simulink model "PIFilter"  (R2024b)
settings: Solver=VariableStepAuto  StartTime=0.0  StopTime=0.5  FixedStep=1e9  RelTol=1e-3
values from neighbouring files (symbols this model uses):
  params = struct()    [initialize_noise_parameters.m]
libraries: fl_lib x19, ee_lib x6, nesl_utility x6
settings Model: Creator=const  LastModifiedBy=const
settings SolverCC: ZeroCrossAlgorithm=Adaptive

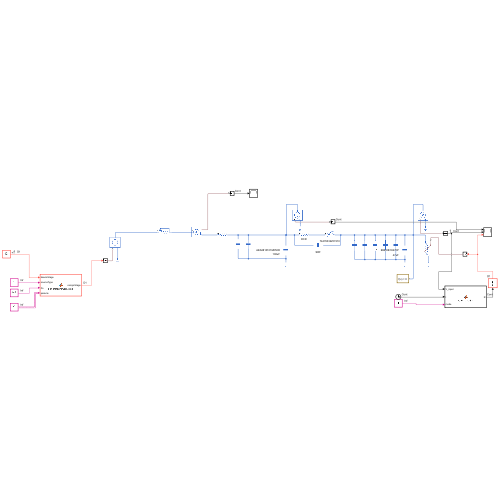
[thumbnail: Simulink's stored preview of the top-level diagram]
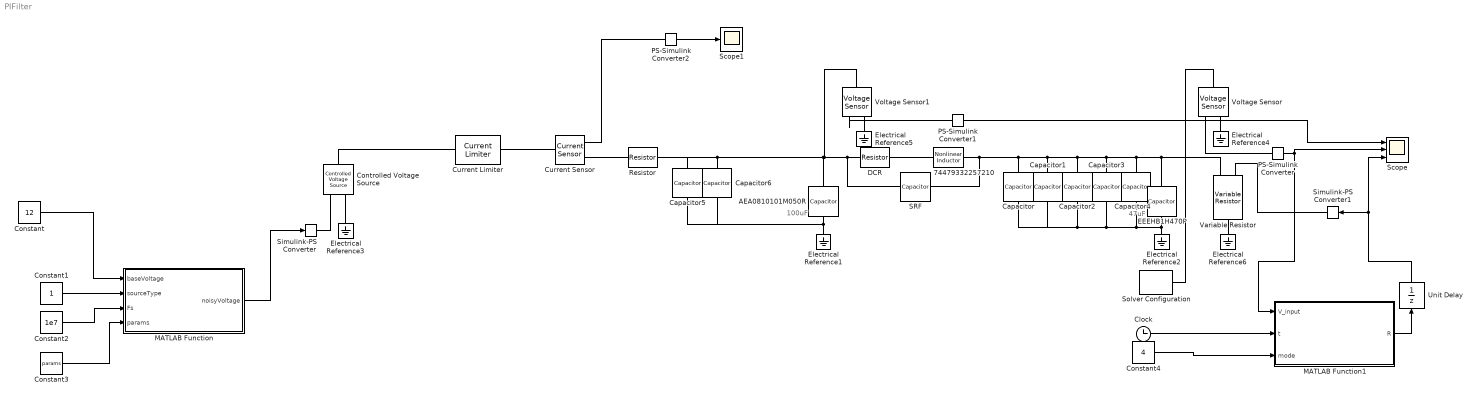
== system PIFilter ==
  note: 100uF
  note: 47uF
  74479332257210 : ee_lib/Passive/Nonlinear Inductor  parameterization_option=3  Nw=10  L=2e-4 H  L_sat=1e-4 H  current_data=[0, 2, 4, 6, 8, 10] A  magnetic_flux_data=[0, 2, 3.95, 5.75, 7.35, 8.77] .* 1e-5 Wb  H_data=[0, 200, 400, 600, 800, 1000] A/m  B_data=[0, .81, 1.25, 1.42, 1.48, 1.49] T  magnetic_flux_sat=1.3e-05 Wb  length_effective=0.032 m  area_effective=1.6e-5 m^2  dBdH0=0.005 T*m/A  B1=1.49 T  H1=1000 A/m  c=0.1  K=200 A/m  alpha=1e-4  averaging_period=0 s  G_parasitic=1e-9 1/Ohm  interpolation_option=1  x0_option=1  i_L0=0 A  phi0=0 Wb  B0=0 T  H0=0 A/m
      settings: InternalSimscapePortConfiguration="{\"Bottom\":[],\"Left\":[{\"id\":\"p\",\"label\":\"+\",\"type\":\"foundation.electrical.electrical\"}],\"Right\":[{\"id\":\"n\",\"label\":\"-\",\"type\":\"foundation.electrical.electrical\"}],\"Top\":[]}"
  AEA0810101M050R : ee_lib/Passive/Capacitor  cap_option=ee.enum.passive.capacitor.capOption.const  c=100e-6 F  Cvec=[1e-05, 1e-06] F  Vvec=[0, 10] V  CV_table_symmetry=ee.enum.passive.capacitor.tableSymmetry.yes  f_vec=[1, 10] kHz  DFext_vec=[.8, 1.2]  enable_C_tol=ee.enum.toleranceApplication.applyRand  averaging_period=0 s  C_tol=20  tol_distribution=ee.enum.toleranceDistribution.uniform  nSigma=4  r=0.34 Ohm  g=1e-6 1/Ohm  enable_operating_limits=ee.enum.enable.yes  operating_limit_action=ee.enum.passive.reportOpLim.warn  max_working_voltage_range=[0, 50] V  power_rating=0.037 W  maxTemperature=105 degC  thermalEnable=false  thermalMass=1 J/K  fault_action=simscape.enum.assert.action.none  t_fault=1 s  i_specify=off  i_priority=None  i=0 A  i_nominal_specify=off  i_nominal_value=1  i_nominal_unit=A  v_specify=off  v_priority=None  v=0 V  v_nominal_specify=off  v_nominal_value=1  v_nominal_unit=V  vc_specify=off  vc_priority=High  vc=0 V  vc_nominal_specify=off  vc_nominal_value=1  vc_nominal_unit=V  T_specify=off  T_priority=None  T=298.15 K  T_nominal_specify=off  T_nominal_value=1  T_nominal_unit=K
  Capacitor{,1..2,5..6} (5 alike) : fl_lib/Electrical/Electrical Elements/Capacitor  c=10 uF  r=1e-6 Ohm  g=0 1/Ohm  i_specify=off  i_priority=None  i=0 A  i_nominal_specify=off  i_nominal_value=1  i_nominal_unit=A  v_specify=off  v_priority=None  v=0 V  v_nominal_specify=off  v_nominal_value=1  v_nominal_unit=V  vc_specify=off  vc_priority=High  vc=0 V  vc_nominal_specify=off  vc_nominal_value=1  vc_nominal_unit=V
  Capacitor3 : fl_lib/Electrical/Electrical Elements/Capacitor  c=4.7 uF  r=1e-6 Ohm  g=0 1/Ohm  i_specify=off  i_priority=None  i=0 A  i_nominal_specify=off  i_nominal_value=1  i_nominal_unit=A  v_specify=off  v_priority=None  v=0 V  v_nominal_specify=off  v_nominal_value=1  v_nominal_unit=V  vc_specify=off  vc_priority=High  vc=0 V  vc_nominal_specify=off  vc_nominal_value=1  vc_nominal_unit=V
  Capacitor4 : fl_lib/Electrical/Electrical Elements/Capacitor  c=2.2 uF  r=1e-6 Ohm  g=0 1/Ohm  i_specify=off  i_priority=None  i=0 A  i_nominal_specify=off  i_nominal_value=1  i_nominal_unit=A  v_specify=off  v_priority=None  v=0 V  v_nominal_specify=off  v_nominal_value=1  v_nominal_unit=V  vc_specify=off  vc_priority=High  vc=0 V  vc_nominal_specify=off  vc_nominal_value=1  vc_nominal_unit=V
  Clock : Clock
  Constant : Constant  Value=12  SampleTime=1e-6
  Constant1 : Constant
  Constant2 : Constant  Value=1e7
  Constant3 : Constant  Value=params  OutDataTypeStr=Bus: paramsBus
  Constant4 : Constant  Value=4
  Controlled Voltage Source : fl_lib/Electrical/Electrical Sources/Controlled Voltage Source
  Current Limiter : ee_lib/Semiconductors & Converters/Current Limiter  limType=ee.enum.semiconductors.currLimType.constLim  iLim=3 A  iLimReverse=1 A  vLim=0.01 V  gLim=1e-3 1/Ohm  thermal_mass=100 J/K  temperature_specify=off  temperature_priority=High  temperature=298.15 K  temperature_nominal_specify=off  temperature_nominal_value=1  temperature_nominal_unit=K
      settings: InternalSimscapePortConfiguration="{\"Bottom\":[],\"Left\":[{\"id\":\"p\",\"label\":\"+\",\"type\":\"foundation.electrical.electrical\"}],\"Right\":[{\"id\":\"n\",\"label\":\"-\",\"type\":\"foundation.electrical.electrical\"}],\"Top\":[]}"
  Current Sensor : fl_lib/Electrical/Electrical Sensors/Current Sensor
  DCR : fl_lib/Electrical/Electrical Elements/Resistor  R=23.3 mOhm  i_specify=off  i_priority=None  i=0 A  i_nominal_specify=off  i_nominal_value=1  i_nominal_unit=A  v_specify=off  v_priority=None  v=0 V  v_nominal_specify=off  v_nominal_value=1  v_nominal_unit=V
  EEEHB1H470P : ee_lib/Passive/Capacitor  cap_option=ee.enum.passive.capacitor.capOption.const  c=47e-6 F  Cvec=[1e-05, 1e-06] F  Vvec=[0, 10] V  CV_table_symmetry=ee.enum.passive.capacitor.tableSymmetry.yes  f_vec=[1, 10] kHz  DFext_vec=[.8, 1.2]  enable_C_tol=ee.enum.toleranceApplication.applyRand  averaging_period=0 s  C_tol=20  tol_distribution=ee.enum.toleranceDistribution.uniform  nSigma=4  r=0.4 Ohm  g=0.47e-6 1/Ohm  enable_operating_limits=ee.enum.enable.yes  operating_limit_action=ee.enum.passive.reportOpLim.warn  max_working_voltage_range=[0, 50] V  power_rating=0.0338 W  maxTemperature=85 degC  thermalEnable=false  thermalMass=1 J/K  fault_action=simscape.enum.assert.action.none  t_fault=1 s  i_specify=off  i_priority=None  i=0 A  i_nominal_specify=off  i_nominal_value=1  i_nominal_unit=A  v_specify=off  v_priority=None  v=0 V  v_nominal_specify=off  v_nominal_value=1  v_nominal_unit=V  vc_specify=off  vc_priority=High  vc=0 V  vc_nominal_specify=off  vc_nominal_value=1  vc_nominal_unit=V  T_specify=off  T_priority=None  T=298.15 K  T_nominal_specify=off  T_nominal_value=1  T_nominal_unit=K
  Electrical Reference{1..6} (6 alike) : fl_lib/Electrical/Electrical Elements/Electrical Reference
  MATLAB Function : MATLAB Function  TreatAsAtomicUnit=on
  MATLAB Function1 : MATLAB Function  TreatAsAtomicUnit=on
  PS-Simulink Converter : nesl_utility/PS-Simulink Converter  PhysicalDomain=network_engine_domain  SubClassName=ps_output  LeftPortType=input  RightPortType=output  PseudoPeriodic=off  Frequencies=[]  VectorFormat=inherit  Unit=inherit  AffineConversion=off
  PS-Simulink Converter1 : nesl_utility/PS-Simulink Converter  PhysicalDomain=network_engine_domain  SubClassName=ps_output  LeftPortType=input  RightPortType=output  PseudoPeriodic=off  Frequencies=[]  VectorFormat=inherit  Unit=inherit  AffineConversion=off
  PS-Simulink Converter2 : nesl_utility/PS-Simulink Converter  PhysicalDomain=network_engine_domain  SubClassName=ps_output  LeftPortType=input  RightPortType=output  PseudoPeriodic=off  Frequencies=[]  VectorFormat=inherit  Unit=inherit  AffineConversion=off
  Resistor : ee_lib/Passive/Resistor  R=30 mOhm  enable_R_tol=ee.enum.toleranceApplication.applyRand  R_tol=1  tol_distribution=ee.enum.toleranceDistribution.uniform  nSigma=4  enable_operating_limits=ee.enum.enable.no  operating_limit_action=ee.enum.passive.reportOpLim.warn  power_rating=1 W  max_working_voltage=100 V  noise_mode=ee.enum.sources.noise.Disabled  Tdevice=25 degC  sample_time=1e-3 s  repeatability=ee.enum.ic.repeatability.notRepeatable  user_seed=0  auto_seed=686172465  fault_action=simscape.enum.assert.action.none  t_fault=1 s  power_derating_T1=70 degC  power_derating_T2=155 degC  operating_temperature_range_vec=[-50, 150] degC  alpha=3.93e-3 1/K  Tmeas=25 degC  thermal_mass=100 J/K  temperature_specify=off  temperature_priority=High  temperature=298.15 K  temperature_nominal_specify=off  temperature_nominal_value=1  temperature_nominal_unit=K
  SRF : ee_lib/Passive/Capacitor  cap_option=ee.enum.passive.capacitor.capOption.const  c=5.6 pF  Cvec=[1e-05, 1e-06] F  Vvec=[0, 10] V  CV_table_symmetry=ee.enum.passive.capacitor.tableSymmetry.yes  f_vec=[1, 10] kHz  DFext_vec=[.8, 1.2]  enable_C_tol=ee.enum.toleranceApplication.none  averaging_period=0 s  C_tol=5  tol_distribution=ee.enum.toleranceDistribution.uniform  nSigma=4  r=0 Ohm  g=0 1/Ohm  enable_operating_limits=ee.enum.enable.no  operating_limit_action=ee.enum.passive.reportOpLim.warn  max_working_voltage_range=[-25, 25] V  power_rating=1 W  maxTemperature=85 degC  thermalEnable=false  thermalMass=1 J/K  fault_action=simscape.enum.assert.action.none  t_fault=1 s  i_specify=off  i_priority=None  i=0 A  i_nominal_specify=off  i_nominal_value=1  i_nominal_unit=A  v_specify=off  v_priority=None  v=0 V  v_nominal_specify=off  v_nominal_value=1  v_nominal_unit=V  vc_specify=off  vc_priority=High  vc=0 V  vc_nominal_specify=off  vc_nominal_value=1  vc_nominal_unit=V  T_specify=off  T_priority=None  T=298.15 K  T_nominal_specify=off  T_nominal_value=1  T_nominal_unit=K
  Scope : Scope  NumInputPorts=3
  Scope1 : Scope
  Simulink-PS Converter : nesl_utility/Simulink-PS Converter  PhysicalDomain=network_engine_domain  SubClassName=ps_input  LeftPortType=input  RightPortType=output  PseudoPeriodic=off  Frequencies=[]  NoiseDistribution=none  NoiseParameters=[]  Unit=1  AffineConversion=off  FilteringAndDerivatives=filter  SimscapeFilterOrder=1  InputFilterTimeConstant=1e-6  UdotUserProvided=0
  Simulink-PS Converter1 : nesl_utility/Simulink-PS Converter  PhysicalDomain=network_engine_domain  SubClassName=ps_input  LeftPortType=input  RightPortType=output  PseudoPeriodic=off  Frequencies=[]  NoiseDistribution=none  NoiseParameters=[]  Unit=1  AffineConversion=off  FilteringAndDerivatives=provide  SimscapeFilterOrder=1  InputFilterTimeConstant=0.001  UdotUserProvided=0
  Solver Configuration : nesl_utility/Solver Configuration  PhysicalDomain=network_engine_domain  SubClassName=solver  LeftPortType=input  RightPortType=generic  Tones=[]  Harmonics=[]  SimulateNoise=off  Profile=off  UseLocalSampling=off  EnableSwitchedLinearOptims=on  FrequencyDomain=off  UseCCode=off  RelTol=0.001  AbsTol=0.001  MinStep=1e-09  ToWorkspace=off  RevertToSquareIcSolve=off  NumHomotopyIterations=100  PhasorMode=off  PhasorModeNumHarmonics=1  ConsistencySolver=NEWTON_XTOL_AFTER_FTOL  IndexReductionMethod=DerivativeReplacement  DoDC=off  ResidualTolerance=1e-09  ConsistencyTolSource=GLOBAL  ConsistencyAbsTol=0.001  ConsistencyRelTol=0.001  ConsistencyTolFactor=0.001  UseLocalSolver=off  LocalSolverChoice=NE_BACKWARD_EULER_ADVANCER  ResolveIndetEquations=on  FunctionEvalNumThread=1  LocalSolverSampleTime=0.001  DoFixedCost=off  MaxNonlinIter=3  MaxModeIter=2  ComputeImpulses=off  ImpulseIterations=2  LinearAlgebra=auto  LinearAlgebraNumThread=0  EquationFormulation=NE_TIME_EF  DelaysMemoryBudget=1024  AutomaticFiltering=on  FilteringTimeConstant=0.001  PartitionStorageMethod=AS_NEEDED  PartitionMemoryBudget=1024  PartitionMethod=ROBUST  MultibodyUseLocalSolver=off  MultibodyLocalSolverChoice=ODE1  MultibodyLocalSolverSampleTime=0.001
  Unit Delay : UnitDelay  SampleTime=-1  HasFrameUpgradeWarning=on
  Variable Resistor : fl_lib/Electrical/Electrical Elements/Variable Resistor  Rmin=1 Ohm  thermalEnable=false  thermal_mass=1 J/K  i_specify=off  i_priority=None  i=0 A  i_nominal_specify=off  i_nominal_value=1  i_nominal_unit=A  v_specify=off  v_priority=None  v=0 V  v_nominal_specify=off  v_nominal_value=1  v_nominal_unit=V  T_specify=off  T_priority=None  T=300 K  T_nominal_specify=off  T_nominal_value=1  T_nominal_unit=K
  Voltage Sensor : fl_lib/Electrical/Electrical Sensors/Voltage Sensor
  Voltage Sensor1 : fl_lib/Electrical/Electrical Sensors/Voltage Sensor
  wires:
  PS-Simulink Converter/1 -> MATLAB Function1/1(V_input), Scope/2
  Constant/1 -> MATLAB Function/1(baseVoltage)
  PS-Simulink Converter1/1 -> Scope/1
  PS-Simulink Converter2/1 -> Scope1/1
  Constant1/1 -> MATLAB Function/2(sourceType)
  Constant2/1 -> MATLAB Function/3(Fs)
  Constant3/1 -> MATLAB Function/4(params)
  MATLAB Function/1(noisyVoltage) -> Simulink-PS Converter/1
  Constant4/1 -> MATLAB Function1/3(mode)
  Clock/1 -> MATLAB Function1/2(t)
  MATLAB Function1/1(R) -> Unit Delay/1
  Unit Delay/1 -> Scope/3, Simulink-PS Converter1/1
  connections:
  DCR/RConn1 -- 74479332257210/LConn1
  EEEHB1H470P/LConn1 -- Solver Configuration/RConn1 -- Variable Resistor/LConn2 -- Voltage Sensor/LConn1 -- Capacitor4/LConn1 -- Capacitor3/LConn1 -- Capacitor2/LConn1 -- Capacitor1/LConn1 -- Capacitor/LConn1 -- SRF/RConn1 -- 74479332257210/RConn1
  Electrical Reference1/LConn1 -- Capacitor6/RConn1 -- Capacitor5/RConn1 -- AEA0810101M050R/RConn1
  Electrical Reference2/LConn1 -- Capacitor4/RConn1 -- Capacitor3/RConn1 -- Capacitor2/RConn1 -- Capacitor1/RConn1 -- Capacitor/RConn1 -- EEEHB1H470P/RConn1
  AEA0810101M050R/LConn1 -- Resistor/RConn1 -- Capacitor5/LConn1 -- Capacitor6/LConn1 -- DCR/LConn1 -- SRF/LConn1 -- Voltage Sensor1/LConn1
  Electrical Reference3/LConn1 -- Controlled Voltage Source/RConn2
  Electrical Reference4/LConn1 -- Voltage Sensor/RConn2
  Electrical Reference5/LConn1 -- Voltage Sensor1/RConn2
  Variable Resistor/RConn1 -- Electrical Reference6/LConn1
  Voltage Sensor/RConn1 -- PS-Simulink Converter/LConn1
  Simulink-PS Converter/RConn1 -- Controlled Voltage Source/RConn1
  Voltage Sensor1/RConn1 -- PS-Simulink Converter1/LConn1
  PS-Simulink Converter2/LConn1 -- Current Sensor/RConn1
  Current Limiter/RConn1 -- Current Sensor/LConn1
  Current Limiter/LConn1 -- Controlled Voltage Source/LConn1
  Simulink-PS Converter1/RConn1 -- Variable Resistor/LConn1
  Current Sensor/RConn2 -- Resistor/LConn1

== matlab function PIFilter/MATLAB Function1 ==
  data: V_input input; R output; t input; mode input
function R = motorLoadSim(V_input, t, mode)
% MOTORLOADSIM Simulink-compatible DC motor load resistance simulator
%
% Inputs:
%   V_input - Supply voltage (V)
%   t       - Current time (seconds) - scalar input from Simulink Clock
%   mode    - Load pattern: 1=steps, 2=triangles, 3=random, 4=mixed
%
% Output:
%   R - Resistance value (ohms) to achieve desired current profile
%
% Motor specs: Max current = 3A

    % Generate current based on mode
    if mode == 1
        % Steps - sharp step changes
        step_levels = [0.3, 1.0, 0.5, 2.0, 0.8, 2.5, 0.4, 3.0];
        step_duration = 0.5;
        idx = floor(t / step_duration) + 1;
        if idx > 8
            idx = mod(idx-1, 8) + 1;
        end
        I_motor = step_levels(idx);
        
    elseif mode == 2
        % Triangles
        freq = 0.5;
        I_min = 0.2;
        I_max = 3.0;
        phase = mod(freq * t, 1.0);
        if phase < 0.5
            I_motor = I_min + (I_max - I_min) * (phase * 2);
        else
            I_motor = I_max - (I_max - I_min) * ((phase - 0.5) * 2);
        end
        
    elseif mode == 3
        % Random-like (deterministic based on time)
        current_levels = [0.3, 0.8, 1.5, 2.2, 2.8, 3.0, 0.5, 1.2];
        idx = floor(mod(t * 3.7, 8)) + 1; % Pseudo-random indexing
        I_motor = current_levels(idx);
        
    else
        % Mixed pattern (mode == 4 or default)
        cycle_time = 20.0; % 20 second full cycle
        t_phase = mod(t, cycle_time) / cycle_time;
        
        if t_phase < 0.25
            % Step pattern
            I_motor = 0.5 + 2.0 * double(mod(t, 0.3) > 0.15);
            
        elseif t_phase < 0.5
            % Triangle
            tri_phase = mod((t_phase - 0.25) * 8, 1.0);
            if tri_phase < 0.5
                I_motor = 0.3 + 2.7 * (tri_phase * 2);
            else
                I_motor = 3.0 - 2.7 * ((tri_phase - 0.5) * 2);
            end
            
        elseif t_phase < 0.75
            % Spikes
            if mod(floor(t * 10), 3) == 0
                I_motor = 3.0;
            else
                I_motor = 0.4;
            end
            
        else
            % Ramp up
            I_motor = 0.3 + 2.7 * ((t_phase - 0.75) / 0.25);
        end
    end
    
    % Clamp current to valid range
    I_motor = max(min(I_motor, 3.0), 0.2);
    
    % Calculate resistance from Ohm's law
    R = V_input / I_motor;
    
    % Clamp resistance to reasonable values
    R = max(min(R, 1000), 0.1);
end

% Simulink Setup Instructions:
% 1. Add MATLAB Function block
% 2. Copy this entire function into the block
% 3. Inputs: V_input (constant), t (from Clock block), mode (constant 1-4)
% 4. Output: R (connect to your varistor model)
% 5. Set Fixed-step solver (e.g., 0.001s for smooth transitions)

== matlab function PIFilter/MATLAB Function ==
  data: baseVoltage input; noisyVoltage output; sourceType input; Fs input; params input
function noisyVoltage = generatePowerNoise(baseVoltage, sourceType, Fs, params)
% generatePowerNoise - Injects realistic electrical noise onto a base voltage signal.
% OPTIMIZED FOR REAL-TIME SIMULINK PERFORMANCE
%
% Syntax:
%   noisyVoltage = generatePowerNoise(baseVoltage, sourceType, Fs, params)
%
% Inputs:
%   baseVoltage - Scalar or vector representing the ideal, noise-free DC voltage.
%   sourceType  - Scalar: 1=usb_pd, 2=li_po, 3=wall_wart, 0=random
%   Fs          - Scalar: Sampling frequency in Hz.
%   params      - Struct: Contains all configurable parameters for each model.
%
% Output:
%   noisyVoltage - Scalar/vector representing the base voltage with noise superimposed.

    % --- Declare extrinsic functions at the top level ---
    coder.extrinsic('fprintf');

    % --- Handle scalar or vector input ---
    isScalar = isscalar(baseVoltage);
    if isScalar
        baseVoltage = baseVoltage(1);
        len = 1;
    else
        len = length(baseVoltage);
    end
    
    % --- Pre-initialize the noise variable ---
    noise = 0;
    
    % --- Convert sourceType to numeric if needed ---
    sourceTypeNum = sourceType;

    % --- Random Source Selection (only once, not every call) ---
    persistent randomSource
    if isempty(randomSource)
        randomSource = 1;
    end
    
    if sourceTypeNum == 0
        sourceTypeNum = randomSource;
        if rand() < 0.01  % Only change source 1% of the time
            randomSource = randi(3);
            fprintf('Switched to source type: %d\n', randomSource);
        end
    end

    % --- Main Dispatcher ---
    if sourceTypeNum == 1
        % USB PD
        noise = generateUsbPdNoise(baseVoltage, Fs, params.usb_pd, len);
    elseif sourceTypeNum == 2
        % Li-Po
        noise = generateLiPoNoise(baseVoltage, Fs, params.li_po, len);
    elseif sourceTypeNum == 3
        % Wall-Wart
        noise = generateWallWartNoise(baseVoltage, Fs, params.wall_wart, len);
    else
        noise = 0;
    end

    % --- Combine base voltage with generated noise ---
    noisyVoltage = baseVoltage + noise;

end

% --- Sub-function for USB PD Noise ---
function noise = generateUsbPdNoise(baseVoltage, Fs, p, len)
    persistent phase_ripple phase_whine hf_state
    
    % Initialize persistent variables
    if isempty(phase_ripple)
        phase_ripple = 0;
        phase_whine = 0;
        hf_state = 0;
    end
    
    dt = 1/Fs;
    
    % Component 1: Simplified High-Frequency Noise (IIR filtered white noise)
    % Much faster than FFT - uses first-order IIR filter
    if Fs >= 2 * 300e6
        white = randn() * sqrt(p.psd_hf * Fs);
        alpha = 0.95; % Filter coefficient for ~100MHz bandwidth approximation
        hf_state = alpha * hf_state + (1-alpha) * white;
        hf_noise = hf_state;
    else
        hf_noise = 0;
    end
    
    % Component 2: Low-Frequency Ripple and Whine (phase accumulator method)
    % Update phases
    phase_ripple = phase_ripple + 2*pi*p.f_sw*dt;
    phase_whine = phase_whine + 2*pi*p.f_whine*dt;
    
    % Wrap phases to [0, 2*pi] to prevent overflow
    phase_ripple = mod(phase_ripple, 2*pi);
    phase_whine = mod(phase_whine, 2*pi);
    
    ripple = (p.V_ripple_pp / 2) * sin(phase_ripple);
    whine = (p.A_whine / 2) * sin(phase_whine);
    
    % Component 3: DC Regulation Error (sample & hold, update slowly)
    persistent dc_offset update_counter
    if isempty(dc_offset)
        dc_offset = 0;
        update_counter = 0;
    end
    
    update_counter = update_counter + 1;
    if update_counter >= Fs * 0.1  % Update every 100ms
        if len == 1
            base_mean = baseVoltage;
        else
            base_mean = baseVoltage(1);  % Use first sample as approximation
        end
        dc_offset = (p.V_reg_percent / 100) * base_mean * (rand() - 0.5) * 2;
        update_counter = 0;
    end

    noise = hf_noise + ripple + whine + dc_offset;
end

% --- Sub-function for Li-Po Battery Noise ---
function noise = generateLiPoNoise(baseVoltage, Fs, p, len)
    persistent en_state bms_phase bms_counter
    
    if isempty(en_state)
        en_state = 0;
        bms_phase = 0;
        bms_counter = 0;
    end
    
    % Component 1: SOC-Dependent Electrochemical Noise (simplified lookup)
    % Approximate V-shape with piecewise linear
    if p.soc < 0.1
        en_std_V = (50 - 40*p.soc/0.1) * 1e-6;
    elseif p.soc < 0.9
        en_std_V = 10e-6;
    else
        en_std_V = (10 + 40*(p.soc-0.9)/0.1) * 1e-6;
    end
    
    % First-order IIR filter for colored noise
    white = randn() * en_std_V;
    alpha = 0.9;
    en_state = alpha * en_state + (1-alpha) * white;
    en_noise = en_state;
    
    % Component 2: ESR voltage sag (DC component)
    esr = p.ESR_base * p.N_series;
    v_sag = p.load_current * esr;
    
    % Component 3: BMS Switching (probabilistic burst)
    bms_noise = 0;
    dt = 1/Fs;
    
    if bms_counter > 0
        % Currently in a burst
        bms_phase = bms_phase + 2*pi*p.f_bms*dt;
        bms_noise = (p.A_bms / 2) * (2*mod(bms_phase/(2*pi), 1) - 1); % Sawtooth approx
        bms_counter = bms_counter - 1;
    else
        % Check if new burst should start
        if rand() < p.P_bms_event
            bms_counter = round(0.001 * Fs); % 1ms burst
            bms_phase = 0;
        end
    end
    
    noise = en_noise + bms_noise - v_sag;
end

% --- Sub-function for Wall-Wart Noise ---
function noise = generateWallWartNoise(baseVoltage, Fs, p, len)
    persistent mode phase_ripple phase_whine jitter_accum switch_counter
    coder.extrinsic('fprintf');
    
    if isempty(mode)
        mode = 1; % 1=linear, 2=smps
        phase_ripple = 0;
        phase_whine = 0;
        jitter_accum = 0;
        switch_counter = 0;
        fprintf('Wall-Wart mode: %d\n', mode);
    end
    
    dt = 1/Fs;
    
    % Switch modes occasionally (every 10 seconds)
    switch_counter = switch_counter + 1;
    if switch_counter >= Fs * 10
        mode = randi(2);
        switch_counter = 0;
        fprintf('Wall-Wart switched to mode: %d\n', mode);
    end
    
    if mode == 1
        % Sub-model A: Unregulated Linear Supply
        phase_ripple = phase_ripple + 2*pi*p.linear.f_ripple*dt;
        phase_ripple = mod(phase_ripple, 2*pi);
        
        ripple = (p.linear.V_ripple_pp / 2) * (2*mod(phase_ripple/(2*pi), 1) - 1); % Sawtooth
        v_droop = p.load_current * p.linear.R_out;
        
        if len == 1
            base_mean = baseVoltage;
        else
            base_mean = baseVoltage(1);
        end
        v_offset = (p.linear.V_no_load_factor - 1) * base_mean;
        
        noise = ripple - v_droop + v_offset;
    else
        % Sub-model B: Low-Cost SMPS
        % Add phase jitter
        jitter_accum = jitter_accum + (p.smps.f_jitter / 100) * randn() * dt;
        phase_ripple = phase_ripple + 2*pi*p.smps.f_sw_unstable*dt + jitter_accum;
        phase_whine = phase_whine + 2*pi*p.smps.f_whine_loud*dt;
        
        phase_ripple = mod(phase_ripple, 2*pi);
        phase_whine = mod(phase_whine, 2*pi);
        
        ripple = (p.smps.V_ripple_smps_pp / 2) * sin(phase_ripple);
        whine = (p.smps.A_whine_loud / 2) * sin(phase_whine);
        noise = ripple + whine;
    end
end
